simulink model "Ethan_MIPI"  (R2025b)
settings: Solver=ode1  StartTime=0.0  StopTime=Ttotal  FixedStep=Tsample  MaxStep=1e-3  RelTol=1e-3
values from neighbouring files (symbols this model uses):
  A_0 = 1.5762    [Para_PV.m]
  alpha_T = 0.048/100    (= 0.00048)    [Para_PV.m]
  beta_T = -0.32/100    (= -0.0032)    [Para_PV.m]
  Cin = Impp_array*(1-D0)/Fsw/delta_Vpv    [Para_DCDC.m]
  delta_x = 0.2    [Para_controller.m]
  Ee = 1    [Para_PV.m]
  Fb = 50    [Para_DCAC.m]
  fmpp = 2e2    (= 200)    [Para_controller.m]
  gamma = -0.0528    [Para_PV.m]
  Iscs = Iscs    (= 8.7)    [Para_PV.m]
  Ki0 = Wn(1)^2/K01/alpha_1    [Para_controller.m]
  Kp = -10    [Para_controller.m]
  Kp0 = (2*Wn(1)*zeta(1)*alpha_1-Wn(1)^2*alpha_2)/K01/alpha_1^2    [Para_controller.m]
  Np = 1    [Para_PV.m]
  Ns = 60    [Para_PV.m]
  qk0 = 11594    [Para_PV.m]
  Tau_d0 = alpha_2/alpha_1    [Para_controller.m]
  Tc = 25    [Para_PV.m]
  Ttotal = 5e-1    (= 0.5)    [Batch_Run_MIPI.m]
  Vdc_ref = 380    [Para_DCAC.m]
  Vmag = 230*sqrt(2)    [Para_DCAC.m]
  Vocs = Vocs/Ns    (= 0.623333333333)    [Para_PV.m]
  x_init = round(Voc_array*.9)    [Para_controller.m]
libraries: slpidlib x1
settings Model: Creator=mwxiao  LastModifiedBy=carter
settings SolverCC: AlgebraicLoopSolver=TrustRegion
settings DataIOCC: LimitDataPoints=on  SaveFormat=Array  SignalLoggingSaveFormat=ModelDataLogs  ReturnWorkspaceOutputs=off  SignalLoggingName=sigsOut
settings OptimizationCC: ExpressionDepthLimit=2147483647.0  LifeSpan=inf
settings DebuggingCC: SaveWithParameterizedLinksMsg=none  UnderspecifiedInitializationDetection=Classic  MergeDetectMultiDrivingBlocksExec=none  SignalResolutionControl=TryResolveAllWithWarning  MultiTaskDSMMsg=warning  MultiTaskCondExecSysMsg=none  FcnCallInpInsideContextMsg=warning  UnconnectedInputMsg=warning  UnconnectedOutputMsg=warning  UnconnectedLineMsg=warning  StateNameClashWarn=warning  SFUnexpectedBacktrackingDiag=warning  SFNoUnconditionalDefaultTransitionDiag=warning  SFExecutionAtInitializationDiag=none  ArithmeticOperatorsInVariantConditions=warning
settings HardwareCC: ProdBitPerPointer=32.0  ProdBitPerSizeT=32.0  ProdBitPerPtrDiffT=32.0  ProdLargestAtomicFloat=None  ProdIntDivRoundTo=Undefined  ProdEndianess=Unspecified  ProdWordSize=32.0  ProdHWDeviceType=32-bit Generic  TargetBitPerPointer=64.0  TargetBitPerSizeT=64.0  TargetBitPerPtrDiffT=64.0  TargetLongLongMode=on  TargetIntDivRoundTo=Zero  TargetEndianess=LittleEndian  TargetWordSize=64.0  TargetHWDeviceType=MATLAB Host  ProdEqTarget=off
settings ModelReferenceCC: EnableRefExpFcnMdlSchedulingChecks=on  PropagateSignalLabelsOutOfModel=off
settings SFSimCC: SimUseLocalCustomCode=off  CustomCodeUndefinedFunction=UseInterfaceOnly
settings RTWCC: RTWUseLocalCustomCode=off  GPUComputeCapability=3.5  DLArmComputeVersion=19.05
settings CodeAppCC: StateflowObjectComments=on
settings GRTTargetCC: TargetLangStandard=C89/C90 (ANSI)  CombineOutputUpdateFcns=off  GRTInterface=on
settings ConfigComp: CovMetricSettings=dw  CovSaveCumulativeToWorkspaceVar=on  CovSaveSingleToWorkspaceVar=on  CovExternalEMLEnable=off

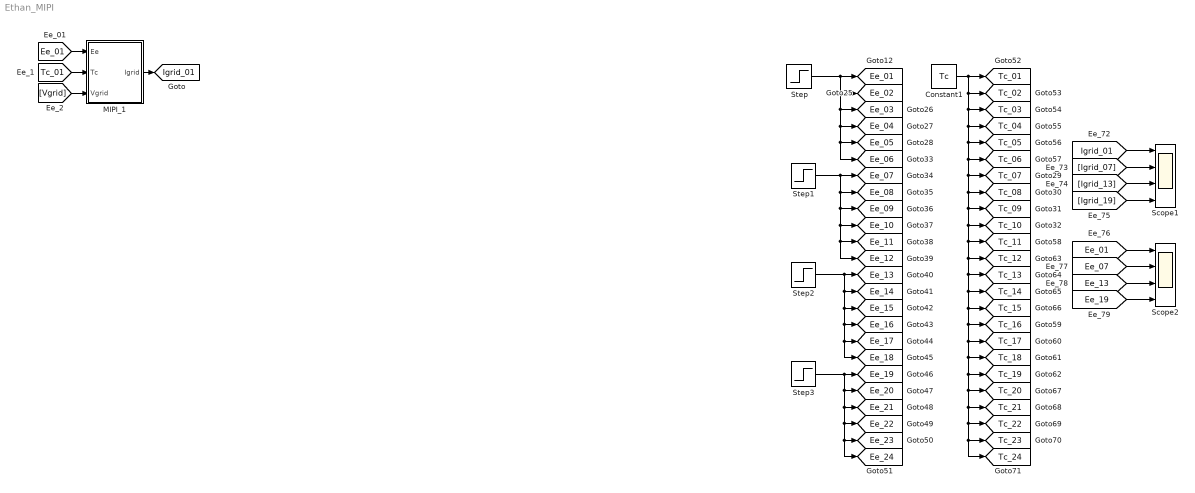
== system Ethan_MIPI ==
  Constant1 : Constant  Value=Tc
  MIPI_1 : Subsystem
  Scope1 : Scope  NumInputPorts=4
      settings: ActiveDisplayYMinimum=-1.5  ActiveDisplayYMaximum=1.5  DataLoggingVariableName=simout
  Scope2 : Scope  NumInputPorts=4
      settings: ActiveDisplayYMinimum=-1.5  ActiveDisplayYMaximum=1.5  DataLoggingVariableName=simout1
  Step : Step  Time=Ttotal/2+0.005  Before=Ee*0.9  After=Ee*0.7  SampleTime=0
  Step1 : Step  Time=Ttotal/2+0.005  Before=Ee*0.8  After=Ee*0.6  SampleTime=0
  Step2 : Step  Time=Ttotal/2+0.005  Before=Ee*0.7  After=Ee*0.5  SampleTime=0
  Step3 : Step  Time=Ttotal/2+0.005  Before=Ee*0.6  After=Ee*0.8  SampleTime=0
  tag scope: Ee_01=global, Ee_02=global, Ee_03=global, Ee_04=global, Ee_05=global, Ee_06=global, Ee_07=global, Ee_08=global, Ee_09=global, Ee_10=global, Ee_11=global, Ee_12=global, Ee_13=global, Ee_14=global, Ee_15=global, Ee_16=global, Ee_17=global, Ee_18=global, Ee_19=global, Ee_20=global, Ee_21=global, Ee_22=global, Ee_23=global, Ee_24=global, Igrid_01=global, Tc_01=global, Tc_02=global, Tc_03=global, Tc_04=global, Tc_05=global, Tc_06=global, Tc_07=global, Tc_08=global, Tc_09=global, Tc_10=global, Tc_11=global, Tc_12=global, Tc_13=global, Tc_14=global, Tc_15=global, Tc_16=global, Tc_17=global, Tc_18=global, Tc_19=global, Tc_20=global, Tc_21=global, Tc_22=global, Tc_23=global, Tc_24=global
  wires:
  [Ee_13] -> Scope2/3
  [Ee_19] -> Scope2/4
  Step1/1 -> [Ee_11], [Ee_12], [Ee_10], [Ee_09], [Ee_08], [Ee_07]
  [Igrid_13] -> Scope1/3
  [Ee_01] -> Scope2/1
  [Igrid_01] -> Scope1/1
  [Igrid_19] -> Scope1/4
  [Ee_07] -> Scope2/2
  [Igrid_07] -> Scope1/2
  Step/1 -> [Ee_01], [Ee_03], [Ee_04], [Ee_05], [Ee_06], [Ee_02]
  Constant1/1 -> [Tc_08], [Tc_17], [Tc_18], [Tc_21], [Tc_22], [Tc_23], [Tc_24], [Tc_20], [Tc_19], [Tc_16], [Tc_15], [Tc_14], [Tc_13], [Tc_12], [Tc_11], [Tc_10], [Tc_09], [Tc_07], [Tc_06], [Tc_05], [Tc_04], [Tc_03], [Tc_02], [Tc_01]
  Step3/1 -> [Ee_23], [Ee_24], [Ee_22], [Ee_21], [Ee_20], [Ee_19]
  Step2/1 -> [Ee_17], [Ee_18], [Ee_16], [Ee_15], [Ee_14], [Ee_13]
  [Vgrid] -> MIPI_1/3(Vgrid)
  [Tc_01] -> MIPI_1/2(Tc)
  [Ee_01] -> MIPI_1/1(Ee)
  MIPI_1/1(Igrid) -> [Igrid_01]

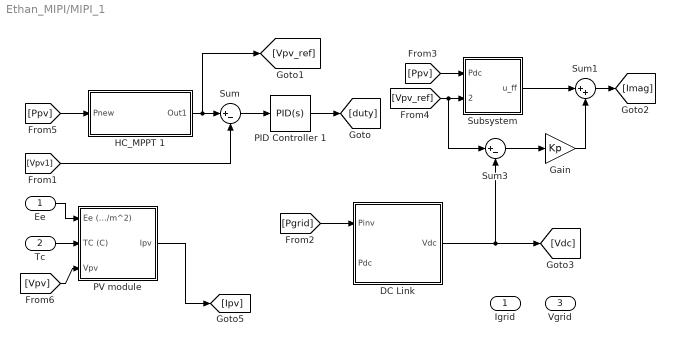
== system Ethan_MIPI/MIPI_1 ==
  Ee : Inport
  Tc : Inport  Port=2
  Vgrid : Inport  Port=3
  DC Link : Subsystem
  Gain : Gain  Gain=Kp
  HC_MPPT 1 : Subsystem
  PID Controller 1 : slpidlib/PID Controller  Controller=PID  Form=Parallel  TimeDomain=Continuous-time  UseExternalTs=off  SampleTime=-1  IntegratorMethod=Forward Euler  FilterMethod=Forward Euler  ControllerParametersSource=internal  P=Kp0  I=Ki0  UseKiTs=off  D=0  UseExternalDerivativeSource=off  N=1/Tau_d0  UseFilter=on  TunerSelectOption=Transfer Function Based (PID Tuner App)  InitialConditionSource=internal  InitialConditionForIntegrator=0  InitialConditionForFilter=0  DifferentiatorICPrevScaledInput=0  ExternalReset=none  TrackingMode=off  Kt=1  LimitOutput=on  SatLimitsSource=internal  UpperSaturationLimit=0.9  LowerSaturationLimit=0  LinearizeAsGain=on  AntiWindupMode=none  Kb=1  LimitIntegrator=off  UpperIntegratorSaturationLimit=inf  LowerIntegratorSaturationLimit=-inf  POutMin=[]  POutMax=[]  IOutMin=[]  IOutMax=[]  DOutMin=[]  DOutMax=[]  NOutMin=[]  NOutMax=[]  SumOutMin=[]  SumOutMax=[]  SaturationOutMin=[]  SaturationOutMax=[]  PParamMin=[]  PParamMax=[]  IParamMin=[]  IParamMax=[]  DParamMin=[]  DParamMax=[]  NParamMin=[]  NParamMax=[]  KbParamMin=[]  KbParamMax=[]  KtParamMin=[]  KtParamMax=[]  KbOutMin=[]  KbOutMax=[]  KtOutMin=[]  KtOutMax=[]  IntegratorOutMin=[]  IntegratorOutMax=[]  FilterOutMin=[]  FilterOutMax=[]  SumI1OutMin=[]  SumI1OutMax=[]  SumI2OutMin=[]  SumI2OutMax=[]  SumI3OutMin=[]  SumI3OutMax=[]  SumI4OutMin=[]  SumI4OutMax=[]  SumDOutMin=[]  SumDOutMax=[]  DifferentiatorOutMin=[]  DifferentiatorOutMax=[]  FilterDiffOutCoefMin=[]  FilterDiffOutCoefMax=[]  ReciprocalOutMin=[]  ReciprocalOutMax=[]  SumDenOutMin=[]  SumDenOutMax=[]  SumNumOutMin=[]  SumNumOutMax=[]  DivideOutMin=[]  DivideOutMax=[]  UdiffTsProdOutMin=[]  UdiffTsProdOutMax=[]  NTsProdOutMin=[]  NTsProdOutMax=[]  UintegralTsProdOutMin=[]  UintegralTsProdOutMax=[]  UngainTsProdOutMin=[]  UngainTsProdOutMax=[]  ClampingZeroOutDataTypeStr=Inherit: Inherit via back propagation  ClampingZeroOutMin=[]  ClampingZeroOutMax=[]  FilterDenConstantOutDataTypeStr=Inherit: Inherit via back propagation  FilterDenConstantOutMin=[]  FilterDenConstantOutMax=[]  PCopyOutDataTypeStr=Inherit: Inherit via back propagation  PCopyOutMin=[]  PCopyOutMax=[]  NCopyOutDataTypeStr=Inherit: Inherit via back propagation  NCopyOutMin=[]  NCopyOutMax=[]  IntegratorContinuousStateAttributes=''  IntegratorStateMustResolveToSignalObject=off  IntegratorRTWStateStorageClass=Auto  FilterContinuousStateAttributes=''  FilterStateMustResolveToSignalObject=off  FilterRTWStateStorageClass=Auto  ParallelPVariant=InternalParameters  IdealPVariant=Disabled  IVariant=InternalParameters  DVariant=InternalParameters  IntegratorVariant=Continuous  SatVariant=Enabled  AWVariant=Passthrough  PCopyVariant=Disabled  TRVariant=Disabled  FdbkBlocksVariant=Forward  IdealPFdbkVariant=Disabled  SatFdbkVariant=Disabled  DerivativeFilterVariant=ContFilter  NVariant=InternalParameters  NCopyVariant=Disabled  FilterICVariant=InternalICsFilter  IntegratorICVariant=InternalICs  ExternalResetVariant=Disabled  TRSumVariant=Passthrough  SumFdbkVariant=Disabled  SumVariant=Sum_PID  TsampFilterVariant=InternalTs  TsampNgainVariant=Passthrough  TsampIntegralVariant=Disabled_SignalSpec  ExternalSaturationOutDataTypeStr=Inherit: Same as second input  DerivativeSourceVariant=ErrorSignal  PreIntVariant=InternalPreInt
  PV module : Subsystem
  Subsystem : Subsystem
  Sum : Sum  Inputs=|+-
  Sum1 : Sum  Inputs=|++
  Sum3 : Sum  Inputs=|+-
  Igrid : Outport
  wires:
  [Vpv] -> PV module/3(Vpv)
  PV module/1(Ipv) -> [Ipv]
  Ee/1 -> PV module/1(Ee (1kW/m^2))
  Tc/1 -> PV module/2(TC (C))
  [Ppv] -> HC_MPPT 1/1(Pnew)
  Sum/1 -> PID Controller 1/1
  PID Controller 1/1 -> [duty]
  [Vpv1] -> Sum/2
  HC_MPPT 1/1(Out1) -> [Vpv_ref], Sum/1
  [Pgrid] -> DC Link/1(Pinv)
  Subsystem/1(u_ff) -> Sum1/1
  Sum3/1 -> Gain/1
  Gain/1 -> Sum1/2
  Sum1/1 -> [Imag]
  [Ppv] -> Subsystem/1(Pdc)
  [Vpv_ref] -> Sum3/1, Subsystem/2(Vdc_ref)
  DC Link/1(Vdc) -> Sum3/2, [Vdc]

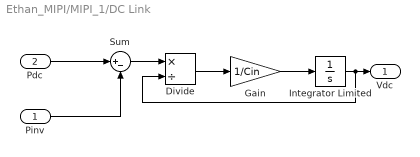
== system Ethan_MIPI/MIPI_1/DC Link ==
  Pinv : Inport
  Pdc : Inport  Port=2
  Divide : Product  Inputs=*/
  Gain : Gain  Gain=1/Cin
  Integrator Limited : Integrator  InitialCondition=Vdc_ref  LimitOutput=on  LowerSaturationLimit=0
  Sum : Sum  Inputs=|+-
  Vdc : Outport
  wires:
  Pdc/1 -> Sum/1
  Pinv/1 -> Sum/2
  Sum/1 -> Divide/1
  Divide/1 -> Gain/1
  Integrator Limited/1 -> Divide/2, Vdc/1
  Gain/1 -> Integrator Limited/1

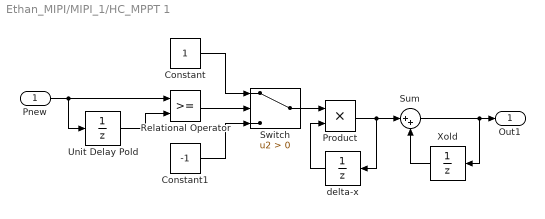
== system Ethan_MIPI/MIPI_1/HC_MPPT 1 ==
  Pnew : Inport  SampleTime=1/fmpp
  Constant : Constant  SampleTime=1/fmpp
  Constant1 : Constant  Value=-1  SampleTime=1/fmpp
  Product : Product
  Relational Operator : RelationalOperator  OutDataTypeStr=boolean  RndMeth=Simplest  InputSameDT=off
  Sum : Sum  Inputs=|++
  Switch : Switch  Criteria=u2 > Threshold  SaturateOnIntegerOverflow=off  InputSameDT=off
  Unit Delay Pold : UnitDelay  InitialCondition=1e3  SampleTime=1/fmpp  HasFrameUpgradeWarning=on
  Xold : UnitDelay  InitialCondition=x_init  SampleTime=1/fmpp  HasFrameUpgradeWarning=on
  delta-x : UnitDelay  InitialCondition=delta_x  SampleTime=1/fmpp  HasFrameUpgradeWarning=on
  Out1 : Outport  SampleTime=1/fmpp
  wires:
  Pnew/1 -> Relational Operator/1, Unit Delay Pold/1
  Unit Delay Pold/1 -> Relational Operator/2
  Relational Operator/1 -> Switch/2
  Constant1/1 -> Switch/3
  Constant/1 -> Switch/1
  Switch/1 -> Product/1
  delta-x/1 -> Product/2
  Product/1 -> Sum/1, delta-x/1
  Sum/1 -> Xold/1, Out1/1
  Xold/1 -> Sum/2

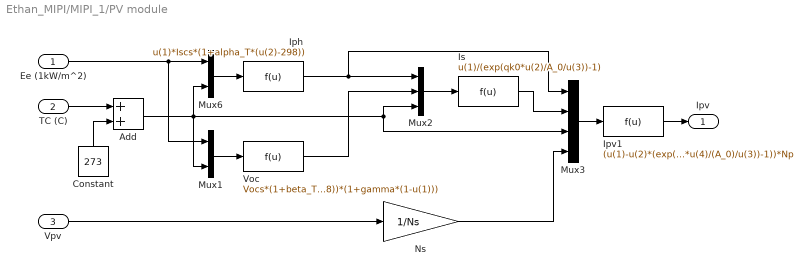
== system Ethan_MIPI/MIPI_1/PV module ==
  Ee (1kW/m^2) : Inport
  TC (C) : Inport  Port=2
  Vpv : Inport  Port=3
  Add : Sum
  Constant : Constant  Value=273
  Iph : Fcn  Expr=u(1)*Iscs*(1+alpha_T*(u(2)-298))
  Ipv1 : Fcn  Expr=(u(1)-u(2)*(exp(qk0*u(4)/(A_0)/u(3))-1))*Np
  Is : Fcn  Expr=u(1)/(exp(qk0*u(2)/A_0/u(3))-1)
  Mux1 : Mux  Inputs=2
  Mux2 : Mux  Inputs=3
  Mux3 : Mux
  Mux6 : Mux  Inputs=2
  Ns : Gain  Gain=1/Ns
  Voc : Fcn  Expr=Vocs*(1+beta_T*(u(2)-298))*(1+gamma*(1-u(1)))
  Ipv : Outport
  wires:
  Mux6/1 -> Iph/1
  Ee (1kW/m^2)/1 -> Mux6/1, Mux1/1
  Mux1/1 -> Voc/1
  Mux2/1 -> Is/1
  Iph/1 -> Mux2/1, Mux3/1
  Voc/1 -> Mux2/2
  Mux3/1 -> Ipv1/1
  Is/1 -> Mux3/2
  Vpv/1 -> Ns/1
  Ipv1/1 -> Ipv/1
  TC (C)/1 -> Add/1
  Add/1 -> Mux6/2, Mux1/2, Mux2/3, Mux3/3
  Constant/1 -> Add/2
  Ns/1 -> Mux3/4

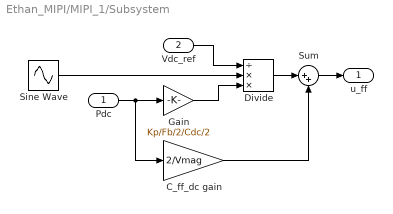
== system Ethan_MIPI/MIPI_1/Subsystem ==
  Pdc : Inport
  Vdc_ref : Inport  Port=2
  C_ff_dc gain : Gain  Gain=2/Vmag
  Divide : Product  Inputs=/**
  Gain : Gain  Gain=Kp/Fb/2/Cdc/2
  Sine Wave : Sin  Amplitude=-1  Frequency=2*pi*Fb*2  SampleTime=0
  Sum : Sum  Inputs=|++
  u_ff : Outport
  wires:
  Pdc/1 -> C_ff_dc gain/1, Gain/1
  Vdc_ref/1 -> Divide/1
  Sine Wave/1 -> Divide/2
  Gain/1 -> Divide/3
  Divide/1 -> Sum/1
  Sum/1 -> u_ff/1
  C_ff_dc gain/1 -> Sum/2
